simulink model "Model"  (R2024b)
settings: Solver=VariableStepAuto  StartTime=0.0  StopTime=10.0  RelTol=1e-3
settings Model: Creator=yugan  LastModifiedBy=sumit
settings RTWCC: GPUComputeCapability=3.5

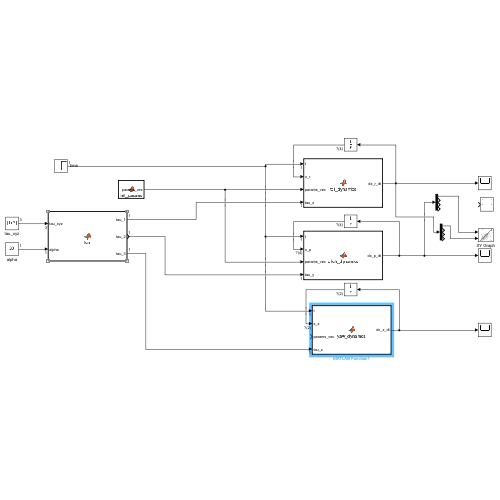
[thumbnail: Simulink's stored preview of the top-level diagram]
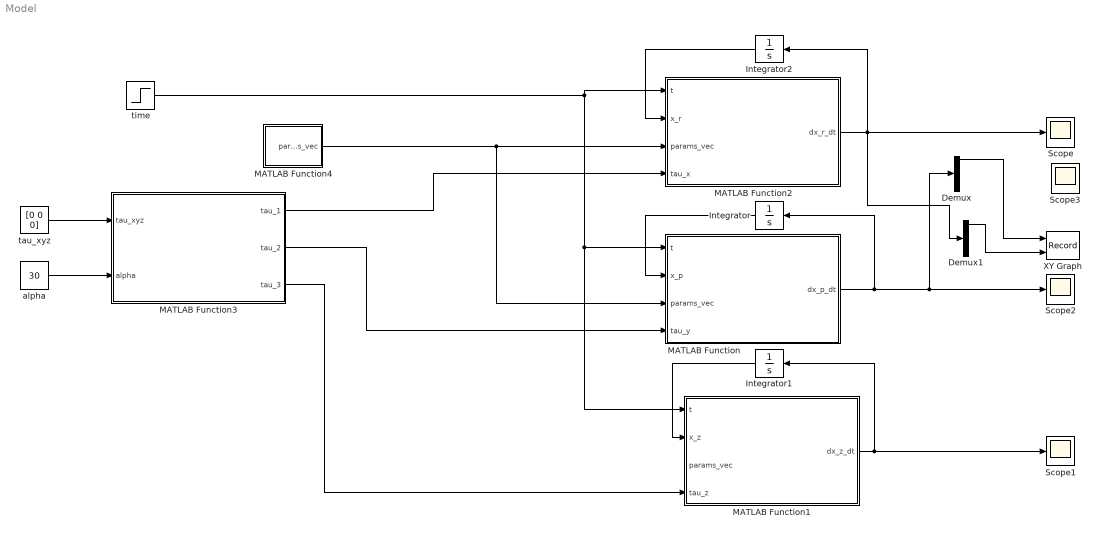
== system Model ==
  Demux : Demux
  Demux1 : Demux
  Integrator : Integrator  InitialCondition=[0; -0.1; 0; 0]
  Integrator1 : Integrator  InitialCondition=[0 ;0]
  Integrator2 : Integrator  InitialCondition=[0; 0.1; 0; 0]
  MATLAB Function : MATLAB Function  TreatAsAtomicUnit=on
  MATLAB Function1 : MATLAB Function  TreatAsAtomicUnit=on
  MATLAB Function2 : MATLAB Function  TreatAsAtomicUnit=on
  MATLAB Function3 : MATLAB Function  TreatAsAtomicUnit=on
  MATLAB Function4 : MATLAB Function  TreatAsAtomicUnit=on
  Scope{,1..3} (4 alike) : Scope
  XY Graph : Record  FileSettingsInternal="{\"entries\":[{\"content\":{\"excelSettings\":{\"content\":{},\"type\":\"Streamout.ExcelSettings\"}},\"type\":\"Streamout.FileSettingStorage\",\"uuid\":\"\"}],\"packageUris\":[\"http:\\/\\/schema.mathworks.com\\/mf0\\/streamout_blocks\\/R2020a\"],\"version\":\"1.0\"}"  Layout=[1 1]  SignalsInternal="{\"entries\":[{\"content\":{\"signals\":[{\"content\":{\"blockPath\":[],\"dimensions\":[1,1],\"domain\":\"\",\"lineColor\":\"#a2142f\",\"plots\":[ 1 ],\"port\":1,\"signalID\":1,\"signalName\":\"Demux:1\"},\"type\":\"RecordBlkView.Signal\",\"uuid\":\"\"},{\"content\":{\"blockPath\":[],\"dimensions\":[1,1],\"domain\":\"\",\"lineColor\":\"#139fff\",\"plots\":[ 1 ],\"port\":2,\"signalID\":2,\"signalName\":\"Demux1:1\"},\"type\":\"RecordBlkView.Signal\",\"uuid\":\"\"}]},\"type\":\"RecordBlkView.InputSignals\",\"uuid\":\"\"}],\"packageUris\":[\"http:\\/\\/schema.mathworks.com\\/mf0\\/streamout_blocks\\/R2020a\"],\"version\":\"1.0\"}"  VisualizationBindings="{\"xyplotplugin\":{\"info\":[{\"series\":[{\"bindingParametersList\":[{\"parameter\":\"X-Axis\",\"signalID\":1,\"signalName\":\"Demux:1\"},{\"parameter\":\"Y-Axis\",\"signalID\":2,\"signalName\":\"Demux1:1\"}],\"seriesID\":0}],\"subplotID\":1}]}}"  CompatibilityTag=XY
  alpha : Constant  Value=30
  tau_xyz : Constant  Value=[0 0 0]
  time : Step  After=10  SampleTime=0
  wires:
  MATLAB Function/1(dx_p_dt) -> Integrator/1, Demux/1, Scope2/1
  Integrator/1 -> MATLAB Function/2(x_p)
  MATLAB Function1/1(dx_z_dt) -> Integrator1/1, Scope1/1
  Integrator1/1 -> MATLAB Function1/2(x_z)
  MATLAB Function2/1(dx_r_dt) -> Demux1/1, Scope/1, Integrator2/1
  Integrator2/1 -> MATLAB Function2/2(x_r)
  alpha/1 -> MATLAB Function3/2(alpha)
  MATLAB Function3/1(tau_1) -> MATLAB Function2/4(tau_x)
  MATLAB Function3/2(tau_2) -> MATLAB Function/4(tau_y)
  MATLAB Function3/3(tau_3) -> MATLAB Function1/4(tau_z)
  time/1 -> MATLAB Function1/1(t), MATLAB Function/1(t), MATLAB Function2/1(t)
  tau_xyz/1 -> MATLAB Function3/1(tau_xyz)
  Demux/1 -> XY Graph/1
  Demux1/1 -> XY Graph/2
  MATLAB Function4/1(params_vec) -> MATLAB Function/3(params_vec), MATLAB Function2/3(params_vec)

== matlab function Model/MATLAB Function1 ==
  data: t input; dx_z_dt output; x_z input; params_vec input; tau_z input
function dx_z_dt = yaw_dynamics(t, x_z, params_vec, tau_z)
% yaw_dynamics.m
%
% 1-DOF yaw dynamic model for Ball Segway.
%
% State x_z = [theta_z ; theta_z_dot]
% params_vec = 20×1 numeric parameter vector (from init_params)
% Output dx_z_dt = state derivative (2×1)

%% ---------------------------------------------------------
% Unpack Parameters From Vector
%% ---------------------------------------------------------

mk  = params_vec(1);     %#ok<NASGU> (not used)
Ik  = params_vec(2);
ma  = params_vec(3);     %#ok<NASGU>
Ix  = params_vec(4);     %#ok<NASGU>
Iy  = params_vec(5);
Iz  = params_vec(6);
l   = params_vec(7);     %#ok<NASGU>
alpha_rad = params_vec(8);
rk  = params_vec(9);
rw  = params_vec(10);
bx  = params_vec(11);    %#ok<NASGU>
dx  = params_vec(12);    %#ok<NASGU>
by  = params_vec(13);    %#ok<NASGU>
dy  = params_vec(14);    %#ok<NASGU>
bry = params_vec(15);    %#ok<NASGU>
dry = params_vec(16);    %#ok<NASGU>
brx = params_vec(17);    %#ok<NASGU>
drx = params_vec(18);    %#ok<NASGU>
g   = params_vec(19);    %#ok<NASGU>
k_motor = params_vec(20); %#ok<NASGU>

% Keep notation same as your original code
I_k_param = Ik;
I_w = Iy;


%% ---------------------------------------------------------
% Extract States
%% ---------------------------------------------------------

theta_z     = x_z(1);
theta_z_dot = x_z(2);


%% ---------------------------------------------------------
% Yaw Dynamics (Eq. 13)
%% ---------------------------------------------------------

num = I_k_param * (rk / rw) * tau_z;

den = I_k_param * Iz + ...
      3 * (I_k_param + Iz) * I_w * (rk / rw)^2 * sin(alpha_rad)^2;

theta_z_ddot = num / den;


%% ---------------------------------------------------------
% Return Derivative
%% ---------------------------------------------------------

dx_z_dt = [ theta_z_dot ;
            theta_z_ddot ];

end

== matlab function Model/MATLAB Function ==
  data: t input; dx_p_dt output; x_p input; params_vec input; tau_y input
function dx_p_dt = pitch_dynamics(t, x_p, params_vec, tau_y)
% pitch_dynamics.m
%
% 2-DOF dynamic model in the X–Z plane (pitch plane).
%
% State x_p = [x_k ; theta_y ; x_k_dot ; theta_y_dot]
% params_vec = 20×1 vector from init_params()
% Output dx_p_dt = state derivative (4×1)

%% ---------------------------------------------------------
% Unpack Parameters from Vector
%% ---------------------------------------------------------

mk  = params_vec(1);     % ball mass
Ik  = params_vec(2);     % ball inertia
ma  = params_vec(3);     % body mass
Ix  = params_vec(4);     % inertia about x
Iy  = params_vec(5);     % inertia about y
Iz  = params_vec(6);     % inertia about z
l   = params_vec(7);     % COM height
alpha_rad = params_vec(8); % zenith angle
rk  = params_vec(9);     % ball radius
rw  = params_vec(10);    % omniwheel radius
bx  = params_vec(11);
dx  = params_vec(12);
by  = params_vec(13);
dy  = params_vec(14);
bry = params_vec(15);
dry = params_vec(16);
brx = params_vec(17);
drx = params_vec(18);
g   = params_vec(19);    % gravity
k_motor = params_vec(20);

% Keep original notation
I_k_param = Ik;
I_w = Iy;    % consistent with roll dynamics formulation


%% ---------------------------------------------------------
% Extract State Variables
%% ---------------------------------------------------------

x_k         = x_p(1);
theta_y     = x_p(2);
x_k_dot     = x_p(3);
theta_y_dot = x_p(4);

q_y_dot = [x_k_dot ; theta_y_dot];


%% ---------------------------------------------------------
% Mass Matrix M(q)   (Eq. 8)
%% ---------------------------------------------------------

M11 = mk + (I_k_param / rk^2) + ma + ...
      (3*I_w*cos(alpha_rad)^2) / (2*rw^2);

M12 =   ma*l*cos(theta_y) ...
      - (3*I_w*cos(alpha_rad)^2)/(2*rw^2) * rk;

M21 = M12;

M22 = ma*l^2 + ...
      (3*I_w*rk^2*cos(alpha_rad)^2)/(2*rw^2) + Iy;

M_y = [M11 M12; M21 M22];


%% ---------------------------------------------------------
% Coriolis–Centrifugal Vector
%% ---------------------------------------------------------

C_y = [ 0                            -ma*l*theta_y_dot*sin(theta_y);
        0                             0 ];


%% ---------------------------------------------------------
% Gravity Vector
%% ---------------------------------------------------------

G_y = [0;
       -ma*g*l*sin(theta_y)];


%% ---------------------------------------------------------
% Friction Vector (ignored)
%% ---------------------------------------------------------

D_y = [0; 0];


%% ---------------------------------------------------------
% Input Torque Vector
%% ---------------------------------------------------------

Q_y = [ -(1/rw) * tau_y ;
         (rk/rw) * tau_y ];


%% ---------------------------------------------------------
% Solve q¨ = M⁻¹ (Q – C q̇ – D – G)
%% ---------------------------------------------------------

q_y_ddot = M_y \ (Q_y - C_y*q_y_dot - D_y - G_y);


%% ---------------------------------------------------------
% Output State Derivatives
%% ---------------------------------------------------------

dx_p_dt = [ x_k_dot ;
            theta_y_dot ;
            q_y_ddot(1) ;
            q_y_ddot(2) ];

end

== matlab function Model/MATLAB Function2 ==
  data: t input; dx_r_dt output; x_r input; params_vec input; tau_x input
function dx_r_dt = roll_dynamics(t, x_r, params_vec, tau_x)
% roll_dynamics.m
%
% State vector x_r = [y_k, theta_x, y_k_dot, theta_x_dot]'

%% 1. Unpack State
y_k         = x_r(1);
theta_x     = x_r(2);
y_k_dot     = x_r(3);
theta_x_dot = x_r(4);
q_x_dot     = [y_k_dot; theta_x_dot];

%% 2. Unpack parameters from vector
mk  = params_vec(1);
Ik  = params_vec(2);
ma  = params_vec(3);
Ix  = params_vec(4);
Iy  = params_vec(5);
Iz  = params_vec(6);
l   = params_vec(7);
alpha_rad = params_vec(8);
rk  = params_vec(9);
rw  = params_vec(10);
bx  = params_vec(11);
dx  = params_vec(12);
by  = params_vec(13);
dy  = params_vec(14);
bry = params_vec(15);
dry = params_vec(16);
brx = params_vec(17);
drx = params_vec(18);
g   = params_vec(19);
k_motor = params_vec(20);

%% 3. Dynamics Matrices (same as original)

% Mass Matrix M(q)
M11 = mk + (Ik / rk^2) + ma + (3*Iy*cos(alpha_rad)^2)/(2*rw^2);
M12 = (3*Iy*cos(alpha_rad)^2)/(2*rw^2)*rk - ma*l*cos(theta_x);
M21 = M12;
M22 = ma*l^2 + (3*Iy*rk^2*cos(alpha_rad)^2)/(2*rw^2) + Ix;
M_x = [M11 M12; M21 M22];

% Coriolis Matrix C(q,q_dot)
C11 = 0;
C12 = ma*l*theta_x_dot*sin(theta_x);
C21 = 0;
C22 = 0;
C_x = [C11 C12; C21 C22];

% Gravity Vector
G1 = 0;
G2 = -ma*g*l*sin(theta_x);
G_x = [G1; G2];

% Friction (optional; currently zero)
D_x = [0; 0];

% Control torque vector
Q1 = (1/rw) * tau_x;
Q2 = (rk/rw) * tau_x;
Q_x = [Q1; Q2];

%% 4. Compute accelerations
q_x_ddot = M_x \ (Q_x - C_x*q_x_dot - D_x - G_x);

%% 5. Output derivative
dx_r_dt = zeros(4,1);
dx_r_dt(1) = y_k_dot;
dx_r_dt(2) = theta_x_dot;
dx_r_dt(3) = q_x_ddot(1);
dx_r_dt(4) = q_x_ddot(2);

end

== matlab function Model/MATLAB Function3 ==
  data: tau_xyz input; tau_1 output; alpha input; tau_2 output; tau_3 output
function [tau_1, tau_2, tau_3] = fcn(tau_xyz, alpha)
% --- Pre-calculate trigonometric terms ---
c_alpha = cos(alpha);
s_alpha = sin(alpha);
sqrt3 = sqrt(3);

% --- Handle potential division by zero ---
% Add a small number (epsilon) to prevent Inf if cos(a) or sin(a) is zero.
if abs(c_alpha) < eps
    c_alpha = sign(c_alpha) * eps; % Keep the sign, but use eps
    if c_alpha == 0 % Handle case where c_alpha was exactly 0
        c_alpha = eps;
    end
end
if abs(s_alpha) < eps
    s_alpha = sign(s_alpha) * eps; % Keep the sign
    if s_alpha == 0 % Handle case where s_alpha was exactly 0
        s_alpha = eps;
    end
end

% --- Define the Matrix M ---
M = [ (2 / (3 * c_alpha)) , 0                    , (1 / (3 * s_alpha));
      (-1 / (3 * c_alpha)), (sqrt3 / (3 * c_alpha)), (1 / (3 * s_alpha));
      (-1 / (3 * c_alpha)), (-sqrt3 / (3 * c_alpha)), (1 / (3 * s_alpha)) ];
      
% --- Perform the matrix multiplication ---
% Ensure tau_xyz is a column vector for correct matrix math
tau_123 = M * tau_xyz(:);

% --- Assign to separate outputs ---
tau_1 = tau_123(1);
tau_2 = tau_123(2);
tau_3 = tau_123(3);

== matlab function Model/MATLAB Function4 ==
  data: params_vec output
function params_vec = init_params()
% init_params.m
% Returns parameters as a 20×1 vector (NO STRUCT)

mk  = 19.6;                   % (1) ball mass
Ik  = 0.38;                   % (2) ball inertia
ma  = 68;                     % (3) body mass
Ix  = 12.1;                   % (4) body inertia x
Iy  = 11.67;                  % (5) body inertia y
Iz  = 1.08;                   % (6) body inertia z
l   = 0.38;                   % (7) COM height
a   = deg2rad(65.5);          % (8) zenith angle
rk  = 0.22;                   % (9) ball radius
rw  = 0.10;                   % (10) omniwheel radius
bx  = 0.10;                   % (11) viscous friction xz
dx  = 0.01;                   % (12) coulomb friction xz
by  = 0.10;                   % (13) viscous friction yz
dy  = 0.01;                   % (14) coulomb friction yz
bry = 0.12;                   % (15) body/ball viscous xz
dry = 0.02;                   % (16) coulomb xz
brx = 0.12;                   % (17) body/ball viscous yz
drx = 0.02;                   % (18) coulomb yz
g   = 9.81;                   % (19) gravity
k_motor = 1;                  % (20) motor constant

% Return as vector
params_vec = [
    mk; Ik; ma; Ix; Iy; Iz;
    l; a; rk; rw;
    bx; dx; by; dy;
    bry; dry; brx; drx;
    g; k_motor
];
end
